simulink model "Zieglerd4_29"  (Simulink 8.3)
settings: Solver=ode45  SolverMode=SingleTasking  StartTime=0.0  StopTime=5  FixedStep=0.001  RelTol=1e-3
values from neighbouring files (symbols this model uses):
  kd = kp*pi/(4*wr)    [ZieglerDm4_29.m]    (also in Zieglerm4_27.m; example4_15.m = 0.01; example4_16.m = 0.006)
  ki = kp*wr/pi    [ZieglerDm4_29.m]    (also in Zieglerm4_27.m; example4_15.m = 1; example4_16.m = 0.01)
  kp = 0.6*kr    [ZieglerDm4_29.m]    (also in Zieglerm4_27.m; example4_15.m = 1.5; example4_16.m = 1.9)
undefined symbols (not defined in the file or in its folder): DiscIntNeverNeededParam
settings Model: Creator=Zhu Supeng  LastModifiedBy=Zhu Supeng  ExtModeTrigMode=oneshot  ExtModeArmWhenConnect=off
settings DataIOCC: LimitDataPoints=off  SignalLoggingName=sigsOut
settings OptimizationCC: BooleanDataType=off
settings DebuggingCC: SaveWithParameterizedLinksMsg=none  SignalResolutionControl=TryResolveAllWithWarning  SolverPrmCheckMsg=none  MultiTaskDSMMsg=warning  MultiTaskCondExecSysMsg=none  StateNameClashWarn=none
settings HardwareCC: TargetUnknown=on
settings RTWCC: IncludeERTFirstTime=on

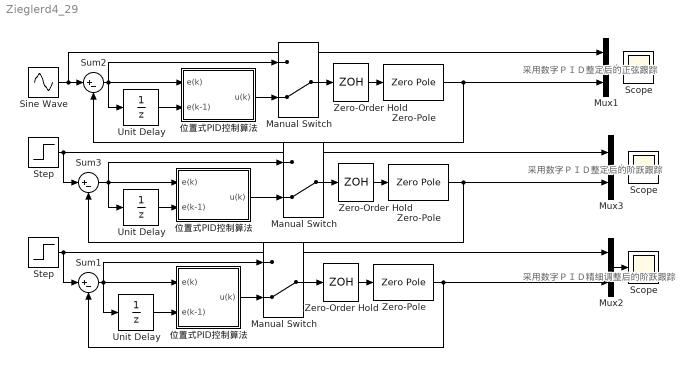
== system Zieglerd4_29 ==
  note: 采用数字ＰＩＤ整定后的正弦跟踪
  note: 采用数字ＰＩＤ整定后的阶跃跟踪
  note: 采用数字ＰＩＤ精细调整后的阶跃跟踪
  " Manual Switch " : ManualSwitch  CurrentSetting=0
  " Scope " : Scope
      settings: YMin=0  YMax=1.2  SaveName=Zieglerdstep1  MaxDataPoints=500000
  " Unit Delay " : UnitDelay  SampleTime=0.1
  " Zero-Order Hold  " : ZeroOrderHold  SampleTime=0.1
  " Zero-Pole " : ZeroPole  Zeros=[]  Poles=[-1 -2]
  " 位置式PID控制算法 " : Subsystem
  Manual Switch : ManualSwitch  CurrentSetting=0
  "Manual Switch " : ManualSwitch  CurrentSetting=0
  Mux1 : Mux  Inputs=2
  Mux2 : Mux  Inputs=2
  Mux3 : Mux  Inputs=2
  Scope : Scope
      settings: YMin=-3.5  YMax=1  SaveName=Zieglerdsine  MaxDataPoints=500000
  "Scope " : Scope
      settings: YMin=-3.5  YMax=1  SaveName=Zieglerdstep  MaxDataPoints=500000
  Sine Wave : Sin  Amplitude=0.5  Frequency=0.05*pi  SampleTime=0
  Step : Step  Time=0  SampleTime=0
  "Step " : Step  Time=0  SampleTime=0
  Sum1 : Sum  Inputs=|+-  SaturateOnIntegerOverflow=on
  Sum2 : Sum  Inputs=|+-  SaturateOnIntegerOverflow=on
  Sum3 : Sum  Inputs=|+-  SaturateOnIntegerOverflow=on
  Unit Delay : UnitDelay  SampleTime=0.1
  "Unit Delay " : UnitDelay  SampleTime=0.1
  Zero-Order Hold : ZeroOrderHold  SampleTime=0.1
  "Zero-Order Hold " : ZeroOrderHold  SampleTime=0.1
  Zero-Pole : ZeroPole  Zeros=[]  Poles=[-1 -2]
  "Zero-Pole " : ZeroPole  Zeros=[]  Poles=[-1 -2]
  "位置式PID控制算法 " : Subsystem
  "位置式PID控制算法  " : Subsystem
  wires:
  Sine Wave/1 -> Sum2/1, Mux1/1
  Mux1/1 -> Scope/1
  Zero-Pole/1 -> Sum2/2, Mux1/2
  Unit Delay/1 -> "位置式PID控制算法  "/2(e(k-1))
  Sum2/1 -> "位置式PID控制算法  "/1(e(k)), Manual Switch/1, Unit Delay/1
  "位置式PID控制算法  "/1(u(k)) -> Manual Switch/2
  Zero-Order Hold/1 -> Zero-Pole/1
  Manual Switch/1 -> Zero-Order Hold/1
  Step/1 -> Sum3/1, Mux3/1
  Mux3/1 -> "Scope "/1
  "Zero-Pole "/1 -> Sum3/2, Mux3/2
  "Unit Delay "/1 -> " 位置式PID控制算法 "/2(e(k-1))
  Sum3/1 -> "Manual Switch "/1, "Unit Delay "/1, " 位置式PID控制算法 "/1(e(k))
  " 位置式PID控制算法 "/1(u(k)) -> "Manual Switch "/2
  "Zero-Order Hold "/1 -> "Zero-Pole "/1
  "Manual Switch "/1 -> "Zero-Order Hold "/1
  "Step "/1 -> Mux2/1, Sum1/1
  Mux2/1 -> " Scope "/1
  " Zero-Pole "/1 -> Mux2/2, Sum1/2
  " Unit Delay "/1 -> "位置式PID控制算法 "/2(e(k-1))
  Sum1/1 -> " Unit Delay "/1, " Manual Switch "/1, "位置式PID控制算法 "/1(e(k))
  "位置式PID控制算法 "/1(u(k)) -> " Manual Switch "/2
  " Zero-Order Hold  "/1 -> " Zero-Pole "/1
  " Manual Switch "/1 -> " Zero-Order Hold  "/1

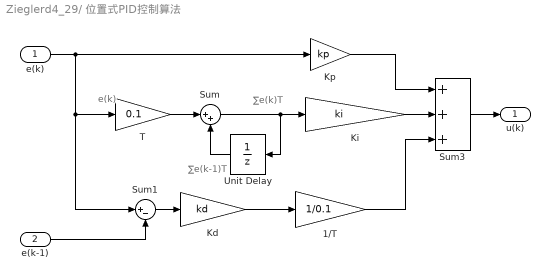
== system Zieglerd4_29/ 位置式PID控制算法  ==
  note: e(k)
  note: ∑e(k)T
  note: ∑e(k-1)T
  e(k) : Inport
  e(k-1) : Inport  Port=2
  1/T : Gain  Gain=1/0.1  SaturateOnIntegerOverflow=on  OutDataTypeStr=Inherit: Same as input  ParamDataTypeStr=Inherit: Same as input
  Kd : Gain  Gain=kd  SaturateOnIntegerOverflow=on  OutDataTypeStr=Inherit: Same as input  ParamDataTypeStr=Inherit: Same as input
  Ki : Gain  Gain=ki  SaturateOnIntegerOverflow=on  OutDataTypeStr=Inherit: Same as input  ParamDataTypeStr=Inherit: Same as input
  Kp : Gain  Gain=kp  SaturateOnIntegerOverflow=on  OutDataTypeStr=Inherit: Same as input  ParamDataTypeStr=Inherit: Same as input
  Sum : Sum  Inputs=|++  SaturateOnIntegerOverflow=on
  Sum1 : Sum  Inputs=|+-  SaturateOnIntegerOverflow=on
  Sum3 : Sum  Inputs=+++  SaturateOnIntegerOverflow=on
  T : Gain  Gain=0.1  SaturateOnIntegerOverflow=on  OutDataTypeStr=Inherit: Same as input  ParamDataTypeStr=Inherit: Same as input
  Unit Delay : UnitDelay  SampleTime=0.1
  u(k) : Outport
  wires:
  e(k-1)/1 -> Sum1/2
  1/T/1 -> Sum3/3
  Kd/1 -> 1/T/1
  Sum3/1 -> u(k)/1
  Ki/1 -> Sum3/2
  Kp/1 -> Sum3/1
  e(k)/1 -> Sum1/1, T/1, Kp/1
  Sum1/1 -> Kd/1
  Sum/1 -> Unit Delay/1, Ki/1
  Unit Delay/1 -> Sum/2
  T/1 -> Sum/1

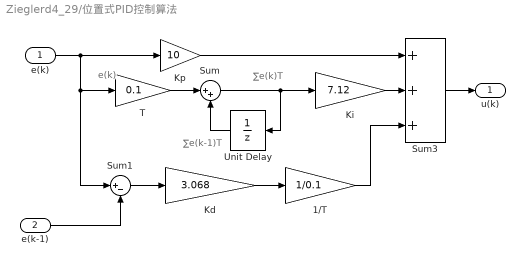
== system Zieglerd4_29/位置式PID控制算法  ==
  note: e(k)
  note: ∑e(k)T
  note: ∑e(k-1)T
  e(k) : Inport
  e(k-1) : Inport  Port=2
  1/T : Gain  Gain=1/0.1  SaturateOnIntegerOverflow=on  OutDataTypeStr=Inherit: Same as input  ParamDataTypeStr=Inherit: Same as input
  Kd : Gain  Gain=3.068  SaturateOnIntegerOverflow=on  OutDataTypeStr=Inherit: Same as input  ParamDataTypeStr=Inherit: Same as input
  Ki : Gain  Gain=7.12  SaturateOnIntegerOverflow=on  OutDataTypeStr=Inherit: Same as input  ParamDataTypeStr=Inherit: Same as input
  Kp : Gain  Gain=10  SaturateOnIntegerOverflow=on  OutDataTypeStr=Inherit: Same as input  ParamDataTypeStr=Inherit: Same as input
  Sum : Sum  Inputs=|++  SaturateOnIntegerOverflow=on
  Sum1 : Sum  Inputs=|+-  SaturateOnIntegerOverflow=on
  Sum3 : Sum  Inputs=+++  SaturateOnIntegerOverflow=on
  T : Gain  Gain=0.1  SaturateOnIntegerOverflow=on  OutDataTypeStr=Inherit: Same as input  ParamDataTypeStr=Inherit: Same as input
  Unit Delay : UnitDelay  SampleTime=0.1
  u(k) : Outport
  wires:
  Sum1/1 -> Kd/1
  e(k)/1 -> Kp/1, Sum1/1, T/1
  Kp/1 -> Sum3/1
  Ki/1 -> Sum3/2
  Sum3/1 -> u(k)/1
  Kd/1 -> 1/T/1
  1/T/1 -> Sum3/3
  Sum/1 -> Unit Delay/1, Ki/1
  Unit Delay/1 -> Sum/2
  e(k-1)/1 -> Sum1/2
  T/1 -> Sum/1

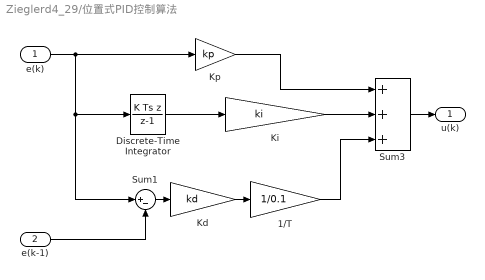
== system Zieglerd4_29/位置式PID控制算法   ==
  e(k) : Inport
  e(k-1) : Inport  Port=2
  1/T : Gain  Gain=1/0.1  SaturateOnIntegerOverflow=on  OutDataTypeStr=Inherit: Same as input  ParamDataTypeStr=Inherit: Same as input
  Discrete-Time Integrator : DiscreteIntegrator  IntegratorMethod=Integration: Backward Euler  SampleTime=0.1  ICPrevOutput=DiscIntNeverNeededParam  ICPrevScaledInput=DiscIntNeverNeededParam
  Kd : Gain  Gain=kd  SaturateOnIntegerOverflow=on  OutDataTypeStr=Inherit: Same as input  ParamDataTypeStr=Inherit: Same as input
  Ki : Gain  Gain=ki  SaturateOnIntegerOverflow=on  OutDataTypeStr=Inherit: Same as input  ParamDataTypeStr=Inherit: Same as input
  Kp : Gain  Gain=kp  SaturateOnIntegerOverflow=on  OutDataTypeStr=Inherit: Same as input  ParamDataTypeStr=Inherit: Same as input
  Sum1 : Sum  Inputs=|+-  SaturateOnIntegerOverflow=on
  Sum3 : Sum  Inputs=+++  SaturateOnIntegerOverflow=on
  u(k) : Outport
  wires:
  e(k-1)/1 -> Sum1/2
  1/T/1 -> Sum3/3
  Kd/1 -> 1/T/1
  Sum3/1 -> u(k)/1
  Ki/1 -> Sum3/2
  Kp/1 -> Sum3/1
  e(k)/1 -> Sum1/1, Discrete-Time Integrator/1, Kp/1
  Sum1/1 -> Kd/1
  Discrete-Time Integrator/1 -> Ki/1
